simulink model "Week2_prob4"  (R2020b)
settings: Solver=VariableStepAuto  StartTime=0.0  StopTime=10  RelTol=1e-3
undefined symbols (not defined in the file): b, J, K, kd, ki, kp, L, R
settings Model: Creator=sai  LastModifiedBy=sai

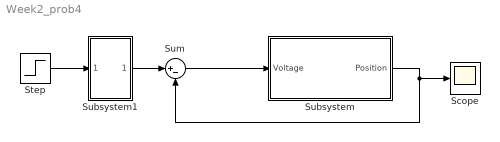
== system Week2_prob4 ==
  Scope : Scope
  Step : Step  SampleTime=0
  Subsystem : Subsystem
  Subsystem1 : Subsystem
  Sum : Sum  Inputs=|+-
  wires:
  Sum/1 -> Subsystem/1(Voltage)
  Subsystem/1(Position) -> Scope/1, Sum/2
  Subsystem1/1(Out1) -> Sum/1
  Step/1 -> Subsystem1/1(In1)

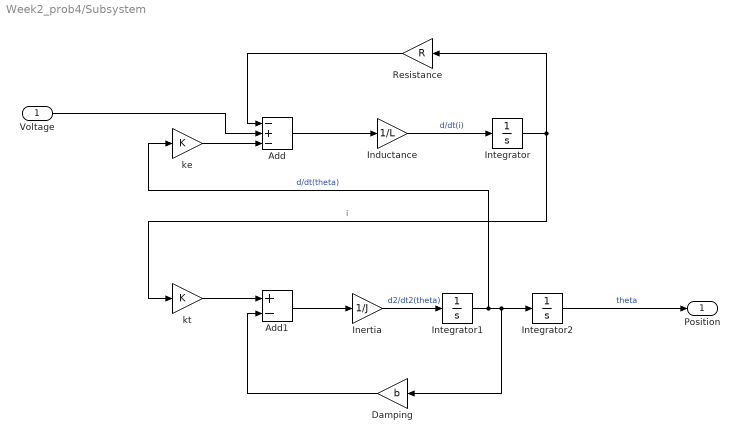
== system Week2_prob4/Subsystem ==
  Voltage : Inport  OutDataTypeStr=double  PortDimensions=1  SampleTime=0
  Add : Sum  Inputs=-+-
  Add1 : Sum  Inputs=+-
  Damping : Gain  Gain=b
  Inductance : Gain  Gain=1/L
  Inertia : Gain  Gain=1/J
  Integrator : Integrator
  Integrator1 : Integrator
  Integrator2 : Integrator
  Resistance : Gain  Gain=R
  ke : Gain  Gain=K
  kt : Gain  Gain=K
  Position : Outport  OutDataTypeStr=double  PortDimensions=1  SampleTime=0
  wires:
  Damping/1 -> Add1/2
  Integrator2/1 -> Position/1  "theta"
  kt/1 -> Add1/1
  Inertia/1 -> Integrator1/1  "d2/dt2(theta)"
  Resistance/1 -> Add/1
  Add/1 -> Inductance/1
  Integrator/1 -> Resistance/1, kt/1  "i"
  Inductance/1 -> Integrator/1  "d/dt(i)"
  Integrator1/1 -> Integrator2/1, Damping/1, ke/1  "d/dt(theta)"
  Voltage/1 -> Add/2
  Add1/1 -> Inertia/1
  ke/1 -> Add/3

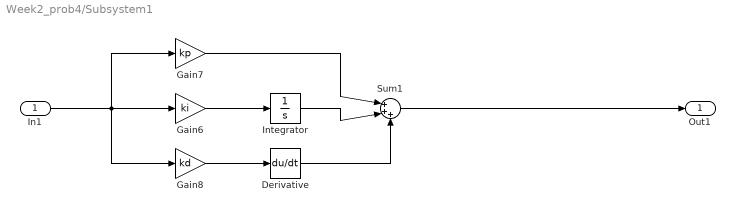
== system Week2_prob4/Subsystem1 ==
  In1 : Inport  OutDataTypeStr=double  PortDimensions=1  SampleTime=0
  Derivative : Derivative
  Gain6 : Gain  Gain=ki
  Gain7 : Gain  Gain=kp
  Gain8 : Gain  Gain=kd
  Integrator : Integrator
  Sum1 : Sum  Inputs=|+++
  Out1 : Outport  OutDataTypeStr=double  PortDimensions=1  SampleTime=0
  wires:
  Gain6/1 -> Integrator/1
  In1/1 -> Gain6/1, Gain7/1, Gain8/1
  Derivative/1 -> Sum1/3
  Integrator/1 -> Sum1/2
  Gain7/1 -> Sum1/1
  Sum1/1 -> Out1/1
  Gain8/1 -> Derivative/1
